simulink model "proba1b"  (Simulink 7.7)
settings: Solver=ode1  StartTime=0.0  StopTime=Inf  FixedStep=0.001  RelTol=1e-3
PostLoadFcn:
  | ,try, rti_mdl_postloadfcn(bdroot, 'UpdateModel', 280, 'rti1005'); catch, disp(lasterr); end,
undefined symbols (not defined in the file or in its folder): ctg, sgn
libraries: simulink x42, simulink_extras x10, rtilibm x8
(part 2 of 2)

== system proba1b/serwomechanizmy/os6/ograniczenie3 ==
  In1 : Inport
  Compare To Constant : simulink/Logic and Bit Operations/Compare To Constant  SystemSampleTime=-1  relop=<=  const=890  LogicOutDataTypeMode=boolean  ZeroCross=off
  Compare To Constant1 : simulink/Logic and Bit Operations/Compare To Constant  SystemSampleTime=-1  relop=>=  const=0  LogicOutDataTypeMode=boolean  ZeroCross=off
  Constant1 : Constant  Value=0
  Logical Operator : Logic  AllPortsSameDT=off  OutDataTypeStr=boolean
  Switch : Switch  Criteria=u2 ~= 0
  Out1 : Outport
  wires:
  In1/1 -> Compare To Constant/1, Compare To Constant1/1, Switch/1
  Compare To Constant1/1 -> Logical Operator/1
  Compare To Constant/1 -> Logical Operator/2
  Logical Operator/1 -> Switch/2
  Constant1/1 -> Switch/3
  Switch/1 -> Out1/1

== system proba1b/serwomechanizmy/os6/skalowanie ==
  In1 : Inport
  Fcn : Fcn  Expr=(u(1)*(2^23)*pi())/1000
  Gain2 : Gain  Gain=1.25/pi()
  Out1 : Outport
  wires:
  Fcn/1 -> Gain2/1
  Gain2/1 -> Out1/1
  In1/1 -> Fcn/1

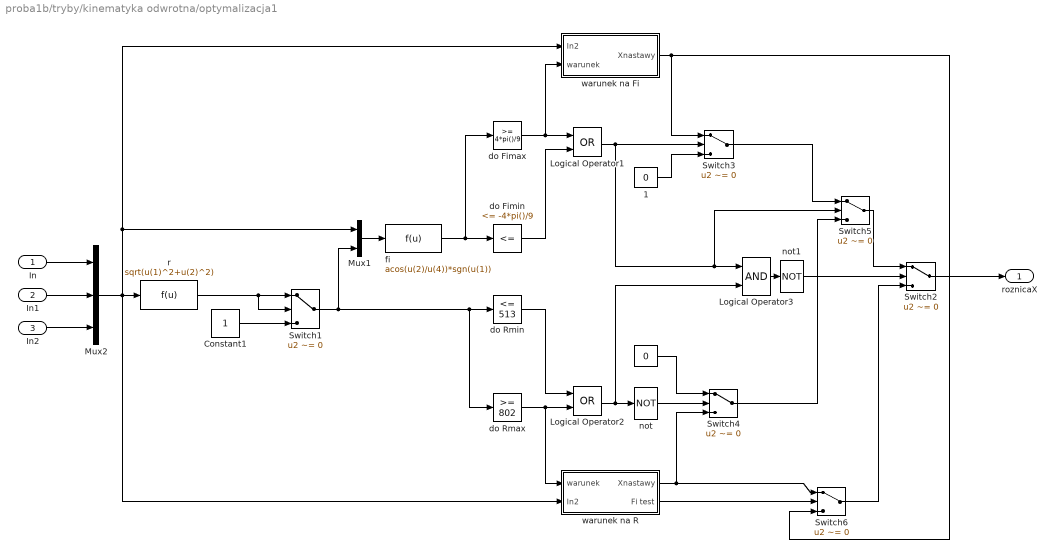
== system proba1b/tryby/kinematyka odwrotna/optymalizacja1 ==
  In : Inport
  In1 : Inport  Port=2
  In2 : Inport  Port=3
  " " : Constant  Value=0  OutDataTypeStr=boolean
  " 1" : Constant  Value=0  OutDataTypeStr=boolean
  Constant1 : Constant  OutDataTypeStr=boolean
  Logical Operator1 : Logic  Operator=OR  AllPortsSameDT=off  OutDataTypeStr=boolean
  Logical Operator2 : Logic  Operator=OR  AllPortsSameDT=off  OutDataTypeStr=boolean
  Logical Operator3 : Logic  AllPortsSameDT=off  OutDataTypeStr=boolean
  Mux1 : Mux  Inputs=2
  Mux2 : Mux  Inputs=3
  Switch{1..6} (6 alike) : Switch  Criteria=u2 ~= 0
  do Fimax : simulink/Logic and Bit Operations/Compare To Constant  SystemSampleTime=-1  relop=>=  const=4*pi()/9  LogicOutDataTypeMode=uint8  ZeroCross=off
  do Fimin : simulink/Logic and Bit Operations/Compare To Constant  SystemSampleTime=-1  relop=<=  const=-4*pi()/9  LogicOutDataTypeMode=uint8  ZeroCross=off
  do Rmax : simulink/Logic and Bit Operations/Compare To Constant  SystemSampleTime=-1  relop=>=  const=802  LogicOutDataTypeMode=uint8  ZeroCross=off
  do Rmin : simulink/Logic and Bit Operations/Compare To Constant  SystemSampleTime=-1  relop=<=  const=513  LogicOutDataTypeMode=uint8  ZeroCross=off
  fi : Fcn  Expr=acos(u(2)/u(4))*sgn(u(1))
  not : Logic  Operator=NOT  AllPortsSameDT=off  OutDataTypeStr=boolean
  not1 : Logic  Operator=NOT  AllPortsSameDT=off  OutDataTypeStr=boolean
  r : Fcn  Expr=sqrt(u(1)^2+u(2)^2)
  warunek na Fi : Subsystem  TreatAsAtomicUnit=on
  warunek na R : Subsystem  TreatAsAtomicUnit=on
  roznicaX : Outport
  wires:
  Switch6/1 -> Switch2/3
  warunek na R/2(Fi test) -> Switch6/2
  not1/1 -> Switch2/2
  Switch3/1 -> Switch5/1
  Switch4/1 -> Switch5/3
  Switch5/1 -> Switch2/1
  Logical Operator3/1 -> not1/1
  " 1"/1 -> Switch3/3
  " "/1 -> Switch4/1
  not/1 -> Switch4/2
  warunek na R/1(Xnastawy) -> Switch6/1, Switch4/3
  warunek na Fi/1(Xnastawy) -> Switch3/1, Switch6/3
  Logical Operator1/1 -> Logical Operator3/1, Switch5/2, Switch3/2
  Logical Operator2/1 -> Logical Operator3/2, not/1
  do Rmax/1 -> warunek na R/1(warunek), Logical Operator2/2
  do Rmin/1 -> Logical Operator2/1
  do Fimin/1 -> Logical Operator1/2
  do Fimax/1 -> warunek na Fi/2(warunek), Logical Operator1/1
  fi/1 -> do Fimax/1, do Fimin/1
  Constant1/1 -> Switch1/3
  Mux1/1 -> fi/1
  Switch1/1 -> do Rmax/1, do Rmin/1, Mux1/2
  r/1 -> Switch1/2, Switch1/1
  Mux2/1 -> r/1, Mux1/1, warunek na Fi/1(In2), warunek na R/2(In2)
  In/1 -> Mux2/1
  In1/1 -> Mux2/2
  In2/1 -> Mux2/3
  Switch2/1 -> roznicaX/1

== system proba1b/tryby/kinematyka odwrotna/podaj wyliczone wartosci ==
  ObliczoneFi1 : Inport
  ObliczoneFi2 : Inport  Port=2
  ObliczoneFi3 : Inport  Port=3
  ObliczoneFi4 : Inport  Port=4
  Enable : EnablePort
  Data Store Write : DataStoreWrite  DataStoreName=obliczoneFi1
  Data Store Write1 : DataStoreWrite  DataStoreName=obliczoneFi2
  Data Store Write2 : DataStoreWrite  DataStoreName=obliczoneFi3
  Data Store Write3 : DataStoreWrite  DataStoreName=obliczoneFi3
  wires:
  ObliczoneFi1/1 -> Data Store Write/1
  ObliczoneFi2/1 -> Data Store Write1/1
  ObliczoneFi3/1 -> Data Store Write2/1
  ObliczoneFi4/1 -> Data Store Write3/1

== system proba1b/tryby/rozpoznawanie obrazu/podaj wyliczone wartosci ==
  zadaneX : Inport
  zadaneY : Inport  Port=2
  zadaneZ : Inport  Port=3
  Data Store Write : DataStoreWrite  DataStoreName=ObliczoneX
  Data Store Write1 : DataStoreWrite  DataStoreName=ObliczoneY
  Data Store Write2 : DataStoreWrite  DataStoreName=ObliczoneZ
  wires:
  zadaneX/1 -> Data Store Write/1
  zadaneY/1 -> Data Store Write1/1
  zadaneZ/1 -> Data Store Write2/1

== system proba1b/RTI Data/RTI Data Store/RTI Data Store/RTI Data Store ==
  RTI Data Store : Subsystem
      mask Type: RTI_DATA_STORE
      mask Description:
      | RTI Data Store Block. This block is used by RTI to store internal model dependent data. Deleting this block will result in data loss.
      | 
      | NEVER DELETE, COPY, OR MODIFY THIS BLOCK!
      mask Help:
      | RTI Data Store Block. This block is used by RTI to store internal model dependent data. Deleting this block will result in data loss.
      | 
      | NEVER DELETE, COPY, OR MODIFY THIS BLOCK!
      mask Display: text(0.5, 0.5, ' ', 'HorizontalAlignment', 'center');

== system proba1b/serwomechanizmy/os1/Position 1/Filters 1 ==
  Sin && Cos : Inport
  Analog Butterworth LP Filter : Subsystem  mask(buttap){@1=2*pi*16, @2=1}
      mask prompts: @1 "Cutoff frequency (rad/sec)"; @2 "Order"
      mask help:
      | Analog Butterworth low pass filter.
      |
      | (Requires Signal Processing Toolbox)
      mask init:
      | [z,p,k]=buttap(@2); z=@1*z; p=@1*p; k=real(prod(-p)); [num,den]=zp2tf(z,p,k); w=logspace(log10(@1/10),log10(10*@1),20); h=freqs(num,den,w);
      mask Help: Butterworth low pass filter using MATLAB's butter command.
      mask Display: plot(20*log10(w),20*log10(abs(h)))
  Analog Butterworth LP Filter1 : Subsystem  mask(buttap){@1=2*pi*16, @2=1}
      mask prompts: @1 "Cutoff frequency (rad/sec)"; @2 "Order"
      mask help:
      | Analog Butterworth low pass filter.
      |
      | (Requires Signal Processing Toolbox)
      mask init:
      | [z,p,k]=buttap(@2); z=@1*z; p=@1*p; k=real(prod(-p)); [num,den]=zp2tf(z,p,k); w=logspace(log10(@1/10),log10(10*@1),20); h=freqs(num,den,w);
      mask Help: Butterworth low pass filter using MATLAB's butter command.
      mask Display: plot(20*log10(w),20*log10(abs(h)))
  Demux : Demux  Outputs=2
  Sin : Outport
  Cos : Outport  Port=2
  wires:
  Demux/2 -> Analog Butterworth LP Filter1/1(In1)
  Demux/1 -> Analog Butterworth LP Filter/1(In1)
  Sin && Cos/1 -> Demux/1
  Analog Butterworth LP Filter1/1(Out1) -> Cos/1
  Analog Butterworth LP Filter/1(Out1) -> Sin/1

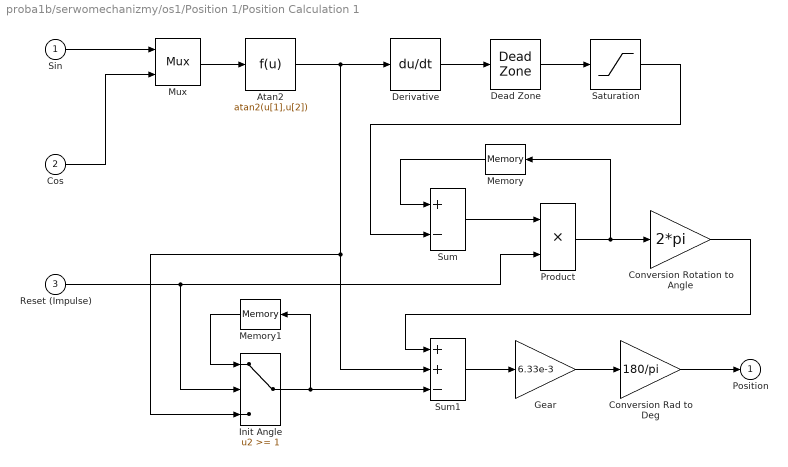
== system proba1b/serwomechanizmy/os1/Position 1/Position Calculation 1 ==
  Sin : Inport
  Cos : Inport  Port=2
  Reset (Impulse) : Inport  Port=3
  Atan2 : Fcn  Expr=atan2(u[1],u[2])
  Conversion Rad to Deg : Gain  Gain=180/pi  SaturateOnIntegerOverflow=on  OutDataTypeStr=Inherit: Same as input  ParamDataTypeStr=Inherit: Same as input
  Conversion Rotation to Angle : Gain  Gain=2*pi  SaturateOnIntegerOverflow=on  OutDataTypeStr=Inherit: Same as input  ParamDataTypeStr=Inherit: Same as input
  Dead Zone : DeadZone  LowerValue=-5000  UpperValue=5000  SaturateOnIntegerOverflow=on
  Derivative : Derivative
  Gear : Gain  Gain=6.33e-3  SaturateOnIntegerOverflow=on  OutDataTypeStr=Inherit: Same as input  ParamDataTypeStr=Inherit: Same as input
  Init Angle : Switch  Threshold=1  SaturateOnIntegerOverflow=on  InputSameDT=on
  Memory : Memory
  Memory1 : Memory
  Mux : Mux  Inputs=2
  Product : Product  SaturateOnIntegerOverflow=on  RndMeth=Zero  InputSameDT=on  OutDataTypeStr=Inherit: Same as first input
  Saturation : Saturate  UpperLimit=1  LowerLimit=-1
  Sum : Sum  Inputs=+-  SaturateOnIntegerOverflow=on  InputSameDT=on  OutDataTypeStr=Inherit: Same as first input
  Sum1 : Sum  Inputs=++-  SaturateOnIntegerOverflow=on  InputSameDT=on  OutDataTypeStr=Inherit: Same as first input
  Position : Outport
  wires:
  Init Angle/1 -> Memory1/1, Sum1/3
  Memory1/1 -> Init Angle/1
  Product/1 -> Memory/1, Conversion Rotation to Angle/1
  Memory/1 -> Sum/1
  Cos/1 -> Mux/2
  Atan2/1 -> Init Angle/3, Sum1/2, Derivative/1
  Reset (Impulse)/1 -> Init Angle/2, Product/2
  Conversion Rotation to Angle/1 -> Sum1/1
  Saturation/1 -> Sum/2
  Conversion Rad to Deg/1 -> Position/1
  Sin/1 -> Mux/1
  Mux/1 -> Atan2/1
  Derivative/1 -> Dead Zone/1
  Dead Zone/1 -> Saturation/1
  Sum/1 -> Product/1
  Sum1/1 -> Gear/1
  Gear/1 -> Conversion Rad to Deg/1

== system proba1b/serwomechanizmy/os1/blok bazowania/zerowanie ==
  Enable : EnablePort
  Constant : Constant  Value=0
  Data Store Write : DataStoreWrite  DataStoreName=u1
  Data Store Write1 : DataStoreWrite  DataStoreName=tmp_u1
  wires:
  Constant/1 -> Data Store Write/1, Data Store Write1/1

== system proba1b/serwomechanizmy/os2/Position 2/Filters 2 ==
  Sin && Cos : Inport
  Analog Butterworth LP Filter : Subsystem  mask(buttap){@1=2*pi*16, @2=1}
      mask prompts: @1 "Cutoff frequency (rad/sec)"; @2 "Order"
      mask help:
      | Analog Butterworth low pass filter.
      |
      | (Requires Signal Processing Toolbox)
      mask init:
      | [z,p,k]=buttap(@2); z=@1*z; p=@1*p; k=real(prod(-p)); [num,den]=zp2tf(z,p,k); w=logspace(log10(@1/10),log10(10*@1),20); h=freqs(num,den,w);
      mask Help: Butterworth low pass filter using MATLAB's butter command.
      mask Display: plot(20*log10(w),20*log10(abs(h)))
  Analog Butterworth LP Filter1 : Subsystem  mask(buttap){@1=2*pi*16, @2=1}
      mask prompts: @1 "Cutoff frequency (rad/sec)"; @2 "Order"
      mask help:
      | Analog Butterworth low pass filter.
      |
      | (Requires Signal Processing Toolbox)
      mask init:
      | [z,p,k]=buttap(@2); z=@1*z; p=@1*p; k=real(prod(-p)); [num,den]=zp2tf(z,p,k); w=logspace(log10(@1/10),log10(10*@1),20); h=freqs(num,den,w);
      mask Help: Butterworth low pass filter using MATLAB's butter command.
      mask Display: plot(20*log10(w),20*log10(abs(h)))
  Demux : Demux  Outputs=2
  Sin : Outport
  Cos : Outport  Port=2
  wires:
  Demux/2 -> Analog Butterworth LP Filter1/1(In1)
  Demux/1 -> Analog Butterworth LP Filter/1(In1)
  Sin && Cos/1 -> Demux/1
  Analog Butterworth LP Filter1/1(Out1) -> Cos/1
  Analog Butterworth LP Filter/1(Out1) -> Sin/1

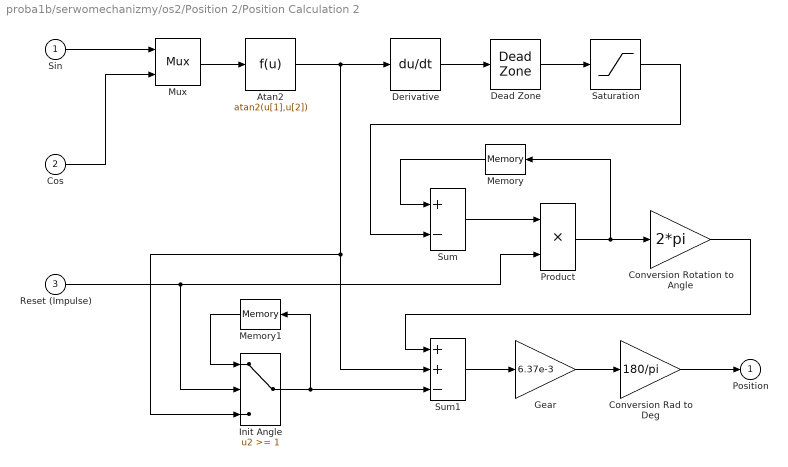
== system proba1b/serwomechanizmy/os2/Position 2/Position Calculation 2 ==
  Sin : Inport
  Cos : Inport  Port=2
  Reset (Impulse) : Inport  Port=3
  Atan2 : Fcn  Expr=atan2(u[1],u[2])
  Conversion Rad to Deg : Gain  Gain=180/pi  SaturateOnIntegerOverflow=on  OutDataTypeStr=Inherit: Same as input  ParamDataTypeStr=Inherit: Same as input
  Conversion Rotation to Angle : Gain  Gain=2*pi  SaturateOnIntegerOverflow=on  OutDataTypeStr=Inherit: Same as input  ParamDataTypeStr=Inherit: Same as input
  Dead Zone : DeadZone  LowerValue=-5000  UpperValue=5000  SaturateOnIntegerOverflow=on
  Derivative : Derivative
  Gear : Gain  Gain=6.37e-3  SaturateOnIntegerOverflow=on  OutDataTypeStr=Inherit: Same as input  ParamDataTypeStr=Inherit: Same as input
  Init Angle : Switch  Threshold=1  SaturateOnIntegerOverflow=on  InputSameDT=on
  Memory : Memory
  Memory1 : Memory
  Mux : Mux  Inputs=2
  Product : Product  SaturateOnIntegerOverflow=on  RndMeth=Zero  InputSameDT=on  OutDataTypeStr=Inherit: Same as first input
  Saturation : Saturate  UpperLimit=1  LowerLimit=-1
  Sum : Sum  Inputs=+-  SaturateOnIntegerOverflow=on  InputSameDT=on  OutDataTypeStr=Inherit: Same as first input
  Sum1 : Sum  Inputs=++-  SaturateOnIntegerOverflow=on  InputSameDT=on  OutDataTypeStr=Inherit: Same as first input
  Position : Outport
  wires:
  Init Angle/1 -> Memory1/1, Sum1/3
  Memory1/1 -> Init Angle/1
  Product/1 -> Memory/1, Conversion Rotation to Angle/1
  Memory/1 -> Sum/1
  Cos/1 -> Mux/2
  Atan2/1 -> Init Angle/3, Sum1/2, Derivative/1
  Reset (Impulse)/1 -> Init Angle/2, Product/2
  Conversion Rotation to Angle/1 -> Sum1/1
  Saturation/1 -> Sum/2
  Conversion Rad to Deg/1 -> Position/1
  Sin/1 -> Mux/1
  Mux/1 -> Atan2/1
  Derivative/1 -> Dead Zone/1
  Dead Zone/1 -> Saturation/1
  Sum/1 -> Product/1
  Sum1/1 -> Gear/1
  Gear/1 -> Conversion Rad to Deg/1

== system proba1b/serwomechanizmy/os2/blok bazowania/zerowanie ==
  Enable : EnablePort
  Constant : Constant  Value=0
  Data Store Write : DataStoreWrite  DataStoreName=u2
  Data Store Write1 : DataStoreWrite  DataStoreName=tmp_u2
  wires:
  Constant/1 -> Data Store Write/1, Data Store Write1/1

== system proba1b/serwomechanizmy/os3/Position 3/Filters 3 ==
  Sin && Cos : Inport
  Analog Butterworth LP Filter : Subsystem  mask(buttap){@1=2*pi*16, @2=1}
      mask prompts: @1 "Cutoff frequency (rad/sec)"; @2 "Order"
      mask help:
      | Analog Butterworth low pass filter.
      |
      | (Requires Signal Processing Toolbox)
      mask init:
      | [z,p,k]=buttap(@2); z=@1*z; p=@1*p; k=real(prod(-p)); [num,den]=zp2tf(z,p,k); w=logspace(log10(@1/10),log10(10*@1),20); h=freqs(num,den,w);
      mask Help: Butterworth low pass filter using MATLAB's butter command.
      mask Display: plot(20*log10(w),20*log10(abs(h)))
  Analog Butterworth LP Filter1 : Subsystem  mask(buttap){@1=2*pi*16, @2=1}
      mask prompts: @1 "Cutoff frequency (rad/sec)"; @2 "Order"
      mask help:
      | Analog Butterworth low pass filter.
      |
      | (Requires Signal Processing Toolbox)
      mask init:
      | [z,p,k]=buttap(@2); z=@1*z; p=@1*p; k=real(prod(-p)); [num,den]=zp2tf(z,p,k); w=logspace(log10(@1/10),log10(10*@1),20); h=freqs(num,den,w);
      mask Help: Butterworth low pass filter using MATLAB's butter command.
      mask Display: plot(20*log10(w),20*log10(abs(h)))
  Demux : Demux  Outputs=2
  Sin : Outport
  Cos : Outport  Port=2
  wires:
  Demux/2 -> Analog Butterworth LP Filter1/1(In1)
  Demux/1 -> Analog Butterworth LP Filter/1(In1)
  Sin && Cos/1 -> Demux/1
  Analog Butterworth LP Filter1/1(Out1) -> Cos/1
  Analog Butterworth LP Filter/1(Out1) -> Sin/1

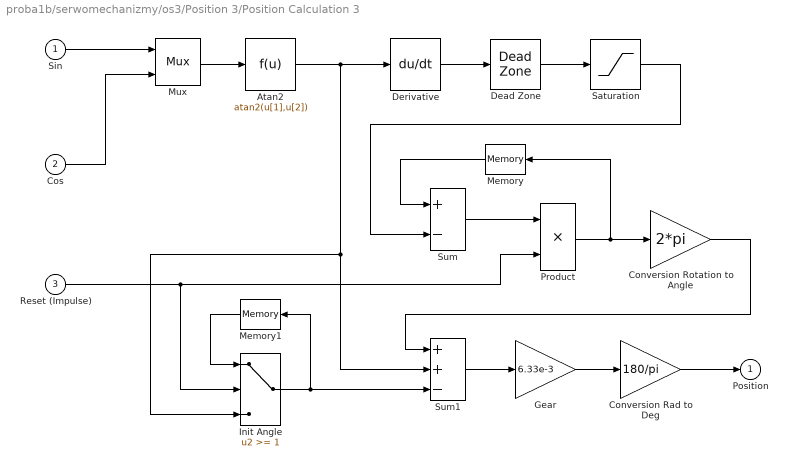
== system proba1b/serwomechanizmy/os3/Position 3/Position Calculation 3 ==
  Sin : Inport
  Cos : Inport  Port=2
  Reset (Impulse) : Inport  Port=3
  Atan2 : Fcn  Expr=atan2(u[1],u[2])
  Conversion Rad to Deg : Gain  Gain=180/pi  SaturateOnIntegerOverflow=on  OutDataTypeStr=Inherit: Same as input  ParamDataTypeStr=Inherit: Same as input
  Conversion Rotation to Angle : Gain  Gain=2*pi  SaturateOnIntegerOverflow=on  OutDataTypeStr=Inherit: Same as input  ParamDataTypeStr=Inherit: Same as input
  Dead Zone : DeadZone  LowerValue=-5000  UpperValue=5000  SaturateOnIntegerOverflow=on
  Derivative : Derivative
  Gear : Gain  Gain=6.33e-3  SaturateOnIntegerOverflow=on  OutDataTypeStr=Inherit: Same as input  ParamDataTypeStr=Inherit: Same as input
  Init Angle : Switch  Threshold=1  SaturateOnIntegerOverflow=on  InputSameDT=on
  Memory : Memory
  Memory1 : Memory
  Mux : Mux  Inputs=2
  Product : Product  SaturateOnIntegerOverflow=on  RndMeth=Zero  InputSameDT=on  OutDataTypeStr=Inherit: Same as first input
  Saturation : Saturate  UpperLimit=1  LowerLimit=-1
  Sum : Sum  Inputs=+-  SaturateOnIntegerOverflow=on  InputSameDT=on  OutDataTypeStr=Inherit: Same as first input
  Sum1 : Sum  Inputs=++-  SaturateOnIntegerOverflow=on  InputSameDT=on  OutDataTypeStr=Inherit: Same as first input
  Position : Outport
  wires:
  Init Angle/1 -> Memory1/1, Sum1/3
  Memory1/1 -> Init Angle/1
  Product/1 -> Memory/1, Conversion Rotation to Angle/1
  Memory/1 -> Sum/1
  Cos/1 -> Mux/2
  Atan2/1 -> Init Angle/3, Sum1/2, Derivative/1
  Reset (Impulse)/1 -> Init Angle/2, Product/2
  Conversion Rotation to Angle/1 -> Sum1/1
  Saturation/1 -> Sum/2
  Conversion Rad to Deg/1 -> Position/1
  Sin/1 -> Mux/1
  Mux/1 -> Atan2/1
  Derivative/1 -> Dead Zone/1
  Dead Zone/1 -> Saturation/1
  Sum/1 -> Product/1
  Sum1/1 -> Gear/1
  Gear/1 -> Conversion Rad to Deg/1

== system proba1b/serwomechanizmy/os3/blok bazowania/zerowanie ==
  Enable : EnablePort
  Constant : Constant  Value=0
  Data Store Write : DataStoreWrite  DataStoreName=u3
  Data Store Write1 : DataStoreWrite  DataStoreName=tmp_u3
  wires:
  Constant/1 -> Data Store Write/1, Data Store Write1/1

== system proba1b/serwomechanizmy/os4/Position 4/Filters 4 ==
  Sin && Cos : Inport
  Analog Butterworth LP Filter : Subsystem  mask(buttap){@1=2*pi*16, @2=1}
      mask prompts: @1 "Cutoff frequency (rad/sec)"; @2 "Order"
      mask help:
      | Analog Butterworth low pass filter.
      |
      | (Requires Signal Processing Toolbox)
      mask init:
      | [z,p,k]=buttap(@2); z=@1*z; p=@1*p; k=real(prod(-p)); [num,den]=zp2tf(z,p,k); w=logspace(log10(@1/10),log10(10*@1),20); h=freqs(num,den,w);
      mask Help: Butterworth low pass filter using MATLAB's butter command.
      mask Display: plot(20*log10(w),20*log10(abs(h)))
  Analog Butterworth LP Filter1 : Subsystem  mask(buttap){@1=2*pi*16, @2=1}
      mask prompts: @1 "Cutoff frequency (rad/sec)"; @2 "Order"
      mask help:
      | Analog Butterworth low pass filter.
      |
      | (Requires Signal Processing Toolbox)
      mask init:
      | [z,p,k]=buttap(@2); z=@1*z; p=@1*p; k=real(prod(-p)); [num,den]=zp2tf(z,p,k); w=logspace(log10(@1/10),log10(10*@1),20); h=freqs(num,den,w);
      mask Help: Butterworth low pass filter using MATLAB's butter command.
      mask Display: plot(20*log10(w),20*log10(abs(h)))
  Demux : Demux  Outputs=2
  Sin : Outport
  Cos : Outport  Port=2
  wires:
  Analog Butterworth LP Filter/1(Out1) -> Sin/1
  Analog Butterworth LP Filter1/1(Out1) -> Cos/1
  Sin && Cos/1 -> Demux/1
  Demux/1 -> Analog Butterworth LP Filter/1(In1)
  Demux/2 -> Analog Butterworth LP Filter1/1(In1)

== system proba1b/serwomechanizmy/os4/Position 4/Position Calculation 4 ==
  Sin : Inport
  Cos : Inport  Port=2
  Reset (Impulse) : Inport  Port=3
  Atan2 : Fcn  Expr=atan2(u[1],u[2])
  Conversion Rad to Deg : Gain  Gain=180/pi  SaturateOnIntegerOverflow=on  OutDataTypeStr=Inherit: Same as input  ParamDataTypeStr=Inherit: Same as input
  Conversion Rotation to Angle : Gain  Gain=2*pi  SaturateOnIntegerOverflow=on  OutDataTypeStr=Inherit: Same as input  ParamDataTypeStr=Inherit: Same as input
  Dead Zone : DeadZone  LowerValue=-5000  UpperValue=5000  SaturateOnIntegerOverflow=on
  Derivative : Derivative
  Gear : Gain  Gain=7.87e-3  SaturateOnIntegerOverflow=on  OutDataTypeStr=Inherit: Same as input  ParamDataTypeStr=Inherit: Same as input
  Init Angle : Switch  Threshold=1  SaturateOnIntegerOverflow=on  InputSameDT=on
  Memory : Memory
  Memory1 : Memory
  Mux : Mux  Inputs=2
  Product : Product  SaturateOnIntegerOverflow=on  RndMeth=Zero  InputSameDT=on  OutDataTypeStr=Inherit: Same as first input
  Saturation : Saturate  UpperLimit=1  LowerLimit=-1
  Sum : Sum  Inputs=+-  SaturateOnIntegerOverflow=on  InputSameDT=on  OutDataTypeStr=Inherit: Same as first input
  Sum1 : Sum  Inputs=++-  SaturateOnIntegerOverflow=on  InputSameDT=on  OutDataTypeStr=Inherit: Same as first input
  Position : Outport
  wires:
  Gear/1 -> Conversion Rad to Deg/1
  Sum1/1 -> Gear/1
  Sum/1 -> Product/1
  Dead Zone/1 -> Saturation/1
  Derivative/1 -> Dead Zone/1
  Mux/1 -> Atan2/1
  Sin/1 -> Mux/1
  Conversion Rad to Deg/1 -> Position/1
  Saturation/1 -> Sum/2
  Conversion Rotation to Angle/1 -> Sum1/1
  Reset (Impulse)/1 -> Product/2, Init Angle/2
  Atan2/1 -> Derivative/1, Sum1/2, Init Angle/3
  Cos/1 -> Mux/2
  Memory/1 -> Sum/1
  Product/1 -> Conversion Rotation to Angle/1, Memory/1
  Memory1/1 -> Init Angle/1
  Init Angle/1 -> Sum1/3, Memory1/1

== system proba1b/serwomechanizmy/os5/Position 5/Filters 5 ==
  Sin && Cos : Inport
  Analog Butterworth LP Filter : Subsystem  mask(buttap){@1=2*pi*16, @2=1}
      mask prompts: @1 "Cutoff frequency (rad/sec)"; @2 "Order"
      mask help:
      | Analog Butterworth low pass filter.
      |
      | (Requires Signal Processing Toolbox)
      mask init:
      | [z,p,k]=buttap(@2); z=@1*z; p=@1*p; k=real(prod(-p)); [num,den]=zp2tf(z,p,k); w=logspace(log10(@1/10),log10(10*@1),20); h=freqs(num,den,w);
      mask Help: Butterworth low pass filter using MATLAB's butter command.
      mask Display: plot(20*log10(w),20*log10(abs(h)))
  Analog Butterworth LP Filter1 : Subsystem  mask(buttap){@1=2*pi*16, @2=1}
      mask prompts: @1 "Cutoff frequency (rad/sec)"; @2 "Order"
      mask help:
      | Analog Butterworth low pass filter.
      |
      | (Requires Signal Processing Toolbox)
      mask init:
      | [z,p,k]=buttap(@2); z=@1*z; p=@1*p; k=real(prod(-p)); [num,den]=zp2tf(z,p,k); w=logspace(log10(@1/10),log10(10*@1),20); h=freqs(num,den,w);
      mask Help: Butterworth low pass filter using MATLAB's butter command.
      mask Display: plot(20*log10(w),20*log10(abs(h)))
  Demux : Demux  Outputs=2
  Sin : Outport
  Cos : Outport  Port=2
  wires:
  Analog Butterworth LP Filter/1(Out1) -> Sin/1
  Analog Butterworth LP Filter1/1(Out1) -> Cos/1
  Sin && Cos/1 -> Demux/1
  Demux/1 -> Analog Butterworth LP Filter/1(In1)
  Demux/2 -> Analog Butterworth LP Filter1/1(In1)

== system proba1b/serwomechanizmy/os5/Position 5/Position Calculation 5 ==
  Sin : Inport
  Cos : Inport  Port=2
  Reset (Impulse) : Inport  Port=3
  Atan2 : Fcn  Expr=atan2(u[1],u[2])
  Conversion Rad to Deg : Gain  Gain=180/pi  SaturateOnIntegerOverflow=on  OutDataTypeStr=Inherit: Same as input  ParamDataTypeStr=Inherit: Same as input
  Conversion Rotation to Angle : Gain  Gain=2*pi  SaturateOnIntegerOverflow=on  OutDataTypeStr=Inherit: Same as input  ParamDataTypeStr=Inherit: Same as input
  Dead Zone : DeadZone  LowerValue=-5000  UpperValue=5000  SaturateOnIntegerOverflow=on
  Derivative : Derivative
  Gear : Gain  Gain=1.32e-2  SaturateOnIntegerOverflow=on  OutDataTypeStr=Inherit: Same as input  ParamDataTypeStr=Inherit: Same as input
  Init Angle : Switch  Threshold=1  SaturateOnIntegerOverflow=on  InputSameDT=on
  Memory : Memory
  Memory1 : Memory
  Mux : Mux  Inputs=2
  Product : Product  SaturateOnIntegerOverflow=on  RndMeth=Zero  InputSameDT=on  OutDataTypeStr=Inherit: Same as first input
  Saturation : Saturate  UpperLimit=1  LowerLimit=-1
  Sum : Sum  Inputs=+-  SaturateOnIntegerOverflow=on  InputSameDT=on  OutDataTypeStr=Inherit: Same as first input
  Sum1 : Sum  Inputs=++-  SaturateOnIntegerOverflow=on  InputSameDT=on  OutDataTypeStr=Inherit: Same as first input
  Position : Outport
  wires:
  Gear/1 -> Conversion Rad to Deg/1
  Sum1/1 -> Gear/1
  Sum/1 -> Product/1
  Dead Zone/1 -> Saturation/1
  Derivative/1 -> Dead Zone/1
  Mux/1 -> Atan2/1
  Sin/1 -> Mux/1
  Conversion Rad to Deg/1 -> Position/1
  Saturation/1 -> Sum/2
  Conversion Rotation to Angle/1 -> Sum1/1
  Reset (Impulse)/1 -> Product/2, Init Angle/2
  Atan2/1 -> Derivative/1, Sum1/2, Init Angle/3
  Cos/1 -> Mux/2
  Memory/1 -> Sum/1
  Product/1 -> Conversion Rotation to Angle/1, Memory/1
  Memory1/1 -> Init Angle/1
  Init Angle/1 -> Sum1/3, Memory1/1

== system proba1b/serwomechanizmy/os6/blok bazowania/zerowanie ==
  Enable : EnablePort
  Constant : Constant  Value=0
  Data Store Write : DataStoreWrite  DataStoreName=u4
  Data Store Write1 : DataStoreWrite  DataStoreName=tmp_u4
  wires:
  Constant/1 -> Data Store Write/1, Data Store Write1/1

== system proba1b/tryby/kinematyka odwrotna/optymalizacja1/warunek na Fi ==
  In2 : Inport
  warunek : Inport  Port=2
  FImax : Constant  Value=4*pi()/9  OutDataTypeStr=boolean
  FImin : Constant  Value=-4*pi()/9  OutDataTypeStr=boolean
  Gain : Gain  Gain=-1
  Mux1 : Mux  Inputs=2
  Mux3 : Mux  Inputs=2
  Subsystem1 : Subsystem
  Subsystem4 : Subsystem
  Switch1 : Switch  Criteria=u2 ~= 0
  Switch4 : Switch  Criteria=u2 ~= 0
  Switch5 : Switch  Criteria=u2 ~= 0
  Xgran : Fcn  Expr=u(2)*ctg(u(4))
  Xnastawy1 : Fcn  Expr=u(1)-u(4)
  Xnastawy2 : Fcn  Expr=u(1)-u(4)
  nieosiagalna : Constant  Value=0  OutDataTypeStr=boolean
  Xnastawy : Outport
  wires:
  Xgran/1 -> Mux3/2
  warunek/1 -> Switch1/2
  FImin/1 -> Switch1/1
  FImax/1 -> Switch1/3
  Switch1/1 -> Mux1/2
  In2/1 -> Mux1/1, Mux3/1
  Mux1/1 -> Xgran/1
  Mux3/1 -> Xnastawy1/1, Gain/1
  Subsystem4/1(Out1) -> Switch4/2
  Switch5/1 -> Switch4/3
  Subsystem1/1(Out1) -> Switch5/2
  nieosiagalna/1 -> Switch5/3
  Switch4/1 -> Xnastawy/1
  Xnastawy1/1 -> Switch4/1, Subsystem4/1(In1)
  Xnastawy2/1 -> Switch5/1, Subsystem1/1(In1)
  Gain/1 -> Xnastawy2/1

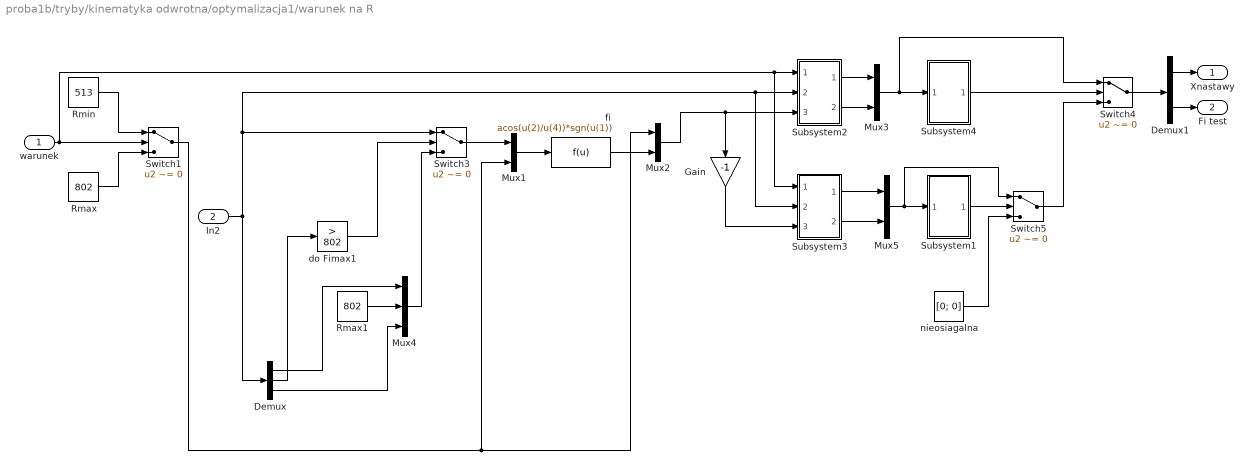
== system proba1b/tryby/kinematyka odwrotna/optymalizacja1/warunek na R ==
  warunek : Inport
  In2 : Inport  Port=2
  Demux : Demux  Outputs=3
  Demux1 : Demux  Outputs=2
  Gain : Gain  Gain=-1
  Mux{1..3,5} (4 alike) : Mux  Inputs=2
  Mux4 : Mux  Inputs=3
  Rmax : Constant  Value=802  OutDataTypeStr=boolean
  Rmax1 : Constant  Value=802  OutDataTypeStr=boolean
  Rmin : Constant  Value=513  OutDataTypeStr=boolean
  Subsystem1 : Subsystem
  Subsystem2 : Subsystem
  Subsystem3 : Subsystem
  Subsystem4 : Subsystem
  Switch{1,3..5} (4 alike) : Switch  Criteria=u2 ~= 0
  do Fimax1 : simulink/Logic and Bit Operations/Compare To Constant  SystemSampleTime=-1  relop=>  const=802  LogicOutDataTypeMode=uint8  ZeroCross=off
  fi : Fcn  Expr=acos(u(2)/u(4))*sgn(u(1))
  nieosiagalna : Constant  Value=[0; 0]  OutDataTypeStr=boolean
  Xnastawy : Outport
  Fi test : Outport  Port=2
  wires:
  fi/1 -> Mux2/2
  Mux1/1 -> fi/1
  In2/1 -> Demux/1, Switch3/1, Subsystem2/2(In2), Subsystem3/2(In2)
  Switch1/1 -> Mux1/2, Mux2/1
  Rmax/1 -> Switch1/3
  Rmin/1 -> Switch1/1
  warunek/1 -> Switch1/2, Subsystem2/1(In1), Subsystem3/1(In1)
  Demux/1 -> Mux4/1
  Demux/3 -> Mux4/3
  Switch3/1 -> Mux1/1
  Demux/2 -> do Fimax1/1
  do Fimax1/1 -> Switch3/2
  Rmax1/1 -> Mux4/2
  Mux4/1 -> Switch3/3
  Subsystem4/1(Out1) -> Switch4/2
  Switch5/1 -> Switch4/3
  Subsystem1/1(Out1) -> Switch5/2
  nieosiagalna/1 -> Switch5/3
  Mux2/1 -> Subsystem2/3(In3), Gain/1
  Demux1/1 -> Xnastawy/1
  Demux1/2 -> Fi test/1
  Switch4/1 -> Demux1/1
  Gain/1 -> Subsystem3/3(In3)
  Mux3/1 -> Switch4/1, Subsystem4/1(In1)
  Subsystem3/1(Out1) -> Mux5/1
  Subsystem3/2(Out2) -> Mux5/2
  Mux5/1 -> Switch5/1, Subsystem1/1(In1)
  Subsystem2/1(Out1) -> Mux3/1
  Subsystem2/2(Out2) -> Mux3/2

== system proba1b/RTI Data/RTI Data Store/RTI Data Store/RTI Data Store/RTI Data Store ==

== system proba1b/serwomechanizmy/os1/Position 1/Filters 1/Analog Butterworth LP Filter ==
  In1 : Inport
  Analog Butterworth LP Filter : ZeroPole  Zeros=z  Poles=p  Gain=k
  Out1 : Outport
  wires:
  Analog Butterworth LP Filter/1 -> Out1/1
  In1/1 -> Analog Butterworth LP Filter/1

== system proba1b/serwomechanizmy/os1/Position 1/Filters 1/Analog Butterworth LP Filter1 ==
  In1 : Inport
  Analog Butterworth LP Filter1 : ZeroPole  Zeros=z  Poles=p  Gain=k
  Out1 : Outport
  wires:
  Analog Butterworth LP Filter1/1 -> Out1/1
  In1/1 -> Analog Butterworth LP Filter1/1

== system proba1b/serwomechanizmy/os2/Position 2/Filters 2/Analog Butterworth LP Filter ==
  In1 : Inport
  Analog Butterworth LP Filter : ZeroPole  Zeros=z  Poles=p  Gain=k
  Out1 : Outport
  wires:
  Analog Butterworth LP Filter/1 -> Out1/1
  In1/1 -> Analog Butterworth LP Filter/1

== system proba1b/serwomechanizmy/os2/Position 2/Filters 2/Analog Butterworth LP Filter1 ==
  In1 : Inport
  Analog Butterworth LP Filter1 : ZeroPole  Zeros=z  Poles=p  Gain=k
  Out1 : Outport
  wires:
  Analog Butterworth LP Filter1/1 -> Out1/1
  In1/1 -> Analog Butterworth LP Filter1/1

== system proba1b/serwomechanizmy/os3/Position 3/Filters 3/Analog Butterworth LP Filter ==
  In1 : Inport
  Analog Butterworth LP Filter : ZeroPole  Zeros=z  Poles=p  Gain=k
  Out1 : Outport
  wires:
  Analog Butterworth LP Filter/1 -> Out1/1
  In1/1 -> Analog Butterworth LP Filter/1

== system proba1b/serwomechanizmy/os3/Position 3/Filters 3/Analog Butterworth LP Filter1 ==
  In1 : Inport
  Analog Butterworth LP Filter1 : ZeroPole  Zeros=z  Poles=p  Gain=k
  Out1 : Outport
  wires:
  Analog Butterworth LP Filter1/1 -> Out1/1
  In1/1 -> Analog Butterworth LP Filter1/1

== system proba1b/serwomechanizmy/os4/Position 4/Filters 4/Analog Butterworth LP Filter ==
  In1 : Inport
  Analog Butterworth LP Filter : ZeroPole  Zeros=z  Poles=p  Gain=k
  Out1 : Outport
  wires:
  Analog Butterworth LP Filter/1 -> Out1/1
  In1/1 -> Analog Butterworth LP Filter/1

== system proba1b/serwomechanizmy/os4/Position 4/Filters 4/Analog Butterworth LP Filter1 ==
  In1 : Inport
  Analog Butterworth LP Filter1 : ZeroPole  Zeros=z  Poles=p  Gain=k
  Out1 : Outport
  wires:
  Analog Butterworth LP Filter1/1 -> Out1/1
  In1/1 -> Analog Butterworth LP Filter1/1

== system proba1b/serwomechanizmy/os5/Position 5/Filters 5/Analog Butterworth LP Filter ==
  In1 : Inport
  Analog Butterworth LP Filter : ZeroPole  Zeros=z  Poles=p  Gain=k
  Out1 : Outport
  wires:
  Analog Butterworth LP Filter/1 -> Out1/1
  In1/1 -> Analog Butterworth LP Filter/1

== system proba1b/serwomechanizmy/os5/Position 5/Filters 5/Analog Butterworth LP Filter1 ==
  In1 : Inport
  Analog Butterworth LP Filter1 : ZeroPole  Zeros=z  Poles=p  Gain=k
  Out1 : Outport
  wires:
  Analog Butterworth LP Filter1/1 -> Out1/1
  In1/1 -> Analog Butterworth LP Filter1/1

== system proba1b/tryby/kinematyka odwrotna/optymalizacja1/warunek na Fi/Subsystem1 ==
  In1 : Inport
  Add : Sum  Inputs=++|
  Aktualne x : DataStoreRead  DataStoreName=u4  SampleTime=0
  Demux1 : Demux  Outputs=2
  Logical Operator4 : Logic  Operator=OR  AllPortsSameDT=off  OutDataTypeStr=boolean
  Mux5 : Mux  Inputs=2
  do Xmax : simulink/Logic and Bit Operations/Compare To Constant  SystemSampleTime=-1  relop=<  const=890  LogicOutDataTypeMode=uint8  ZeroCross=off
  do Xmin : simulink/Logic and Bit Operations/Compare To Constant  SystemSampleTime=-1  relop=>  const=0  LogicOutDataTypeMode=uint8  ZeroCross=off
  Out1 : Outport
  wires:
  Demux1/2 -> Mux5/2
  Demux1/1 -> Add/1
  In1/1 -> Demux1/1
  Mux5/1 -> Out1/1
  Logical Operator4/1 -> Mux5/1
  Add/1 -> do Xmax/1, do Xmin/1
  Aktualne x/1 -> Add/2
  do Xmax/1 -> Logical Operator4/2
  do Xmin/1 -> Logical Operator4/1

== system proba1b/tryby/kinematyka odwrotna/optymalizacja1/warunek na Fi/Subsystem4 ==
  In1 : Inport
  Add : Sum  Inputs=++|
  Aktualne x : DataStoreRead  DataStoreName=u4  SampleTime=0
  Demux1 : Demux  Outputs=2
  Logical Operator4 : Logic  Operator=OR  AllPortsSameDT=off  OutDataTypeStr=boolean
  Mux5 : Mux  Inputs=2
  do Xmax : simulink/Logic and Bit Operations/Compare To Constant  SystemSampleTime=-1  relop=<  const=890  LogicOutDataTypeMode=uint8  ZeroCross=off
  do Xmin : simulink/Logic and Bit Operations/Compare To Constant  SystemSampleTime=-1  relop=>  const=0  LogicOutDataTypeMode=uint8  ZeroCross=off
  Out1 : Outport
  wires:
  do Xmin/1 -> Logical Operator4/1
  do Xmax/1 -> Logical Operator4/2
  Aktualne x/1 -> Add/2
  Add/1 -> do Xmin/1, do Xmax/1
  Logical Operator4/1 -> Mux5/1
  Mux5/1 -> Out1/1
  In1/1 -> Demux1/1
  Demux1/1 -> Add/1
  Demux1/2 -> Mux5/2

== system proba1b/tryby/kinematyka odwrotna/optymalizacja1/warunek na R/Subsystem1 ==
  In1 : Inport
  Add : Sum  Inputs=++|
  Aktualne x : DataStoreRead  DataStoreName=u4  SampleTime=0
  Demux1 : Demux  Outputs=2
  Logical Operator4 : Logic  Operator=OR  AllPortsSameDT=off  OutDataTypeStr=boolean
  Mux5 : Mux  Inputs=2
  do Xmax : simulink/Logic and Bit Operations/Compare To Constant  SystemSampleTime=-1  relop=<  const=890  LogicOutDataTypeMode=uint8  ZeroCross=off
  do Xmin : simulink/Logic and Bit Operations/Compare To Constant  SystemSampleTime=-1  relop=>  const=0  LogicOutDataTypeMode=uint8  ZeroCross=off
  Out1 : Outport
  wires:
  Demux1/2 -> Mux5/2
  Demux1/1 -> Add/1
  In1/1 -> Demux1/1
  Mux5/1 -> Out1/1
  Logical Operator4/1 -> Mux5/1
  Add/1 -> do Xmax/1, do Xmin/1
  Aktualne x/1 -> Add/2
  do Xmax/1 -> Logical Operator4/2
  do Xmin/1 -> Logical Operator4/1

== system proba1b/tryby/kinematyka odwrotna/optymalizacja1/warunek na R/Subsystem2 ==
  In1 : Inport
  In2 : Inport  Port=2
  In3 : Inport  Port=3
  Gain : Gain  Gain=-1
  Logical Operator1 : Logic  Operator=OR  AllPortsSameDT=off  OutDataTypeStr=boolean
  Mux3 : Mux  Inputs=2
  Switch2 : Switch  Criteria=u2 ~= 0
  Xgran : Fcn  Expr=u(1)*sin(u(2))
  Xgran1 : Fcn  Expr=u(1)-u(4)
  do Fimax : simulink/Logic and Bit Operations/Compare To Constant  SystemSampleTime=-1  relop=>=  const=4*pi()/9  LogicOutDataTypeMode=uint8  ZeroCross=off
  do Fimin : simulink/Logic and Bit Operations/Compare To Constant  SystemSampleTime=-1  relop=<=  const=-4*pi()/9  LogicOutDataTypeMode=uint8  ZeroCross=off
  Out1 : Outport
  Out2 : Outport  Port=2
  wires:
  do Fimin/1 -> Logical Operator1/2
  do Fimax/1 -> Logical Operator1/1
  Xgran/1 -> do Fimin/1, do Fimax/1, Mux3/2
  Gain/1 -> Switch2/1
  Xgran1/1 -> Gain/1, Switch2/3
  Mux3/1 -> Xgran1/1
  In2/1 -> Mux3/1
  In1/1 -> Switch2/2
  Switch2/1 -> Out1/1
  In3/1 -> Xgran/1
  Logical Operator1/1 -> Out2/1

== system proba1b/tryby/kinematyka odwrotna/optymalizacja1/warunek na R/Subsystem3 ==
  In1 : Inport
  In2 : Inport  Port=2
  In3 : Inport  Port=3
  Gain : Gain  Gain=-1
  Logical Operator1 : Logic  Operator=OR  AllPortsSameDT=off  OutDataTypeStr=boolean
  Mux3 : Mux  Inputs=2
  Switch2 : Switch  Criteria=u2 ~= 0
  Xgran : Fcn  Expr=u(1)*sin(u(2))
  Xgran1 : Fcn  Expr=u(1)-u(4)
  do Fimax : simulink/Logic and Bit Operations/Compare To Constant  SystemSampleTime=-1  relop=>=  const=4*pi()/9  LogicOutDataTypeMode=uint8  ZeroCross=off
  do Fimin : simulink/Logic and Bit Operations/Compare To Constant  SystemSampleTime=-1  relop=<=  const=-4*pi()/9  LogicOutDataTypeMode=uint8  ZeroCross=off
  Out1 : Outport
  Out2 : Outport  Port=2
  wires:
  Logical Operator1/1 -> Out2/1
  In3/1 -> Xgran/1
  Switch2/1 -> Out1/1
  In1/1 -> Switch2/2
  In2/1 -> Mux3/1
  Mux3/1 -> Xgran1/1
  Xgran1/1 -> Switch2/3, Gain/1
  Gain/1 -> Switch2/1
  Xgran/1 -> Mux3/2, do Fimax/1, do Fimin/1
  do Fimax/1 -> Logical Operator1/1
  do Fimin/1 -> Logical Operator1/2

== system proba1b/tryby/kinematyka odwrotna/optymalizacja1/warunek na R/Subsystem4 ==
  In1 : Inport
  Add : Sum  Inputs=++|
  Aktualne x : DataStoreRead  DataStoreName=u4  SampleTime=0
  Demux1 : Demux  Outputs=2
  Logical Operator4 : Logic  Operator=OR  AllPortsSameDT=off  OutDataTypeStr=boolean
  Mux5 : Mux  Inputs=2
  do Xmax : simulink/Logic and Bit Operations/Compare To Constant  SystemSampleTime=-1  relop=<  const=890  LogicOutDataTypeMode=uint8  ZeroCross=off
  do Xmin : simulink/Logic and Bit Operations/Compare To Constant  SystemSampleTime=-1  relop=>  const=0  LogicOutDataTypeMode=uint8  ZeroCross=off
  Out1 : Outport
  wires:
  do Xmin/1 -> Logical Operator4/1
  do Xmax/1 -> Logical Operator4/2
  Aktualne x/1 -> Add/2
  Add/1 -> do Xmin/1, do Xmax/1
  Logical Operator4/1 -> Mux5/1
  Mux5/1 -> Out1/1
  In1/1 -> Demux1/1
  Demux1/1 -> Add/1
  Demux1/2 -> Mux5/2

== matlab function tryby/rozpoznawanie obrazu/Embedded MATLAB Function ==
  data: x output double; y output double; z output double; k input double
function [x, y, z] = fcn(k)
% This block supports the Embedded MATLAB subset.
% See the help menu for details. 


x = 700+k;
y = 200+k;
z = 1100+k;
